simulink model "penddemo_disc"  (R2021a)
settings: Solver=ode8  StartTime=0  StopTime=inf  FixedStep=0.001  MaxStep=0.02  RelTol=1e-3  AbsTol=1e-6
undefined symbols (not defined in the file or in its folder): DiscIntNeverNeededParam
libraries: cstblocks x1
Description:
  | Inverted Pendulum with Animation
  | 
  | This example shows how to model an inverted pendulum.  The animation is created using MATLAB(R) Handle Graphics(R).  The animation block is a masked
  | S-function.  For more information, use the context menu to look under the Animation block's mask
  | and open the S-function for editing.
settings Model: ExtModeAutoUpdateStatusClock=off  Creator=The MathWorks, Inc.  LastModifiedBy=uidr9910
settings SolverCC: AutoScaleAbsTol=off  AlgebraicLoopSolver=TrustRegion
settings DataIOCC: ExternalInput=[]  InitialState=[]  SaveFormat=Array  SaveOutput=off  SaveTime=off
settings OptimizationCC: BlockReduction=off  BooleanDataType=off  ExpressionDepthLimit=2147483647  InitFltsAndDblsToZero=on  LifeSpan=inf
settings DebuggingCC: SaveWithParameterizedLinksMsg=none  UnderspecifiedInitializationDetection=Classic  MergeDetectMultiDrivingBlocksExec=none  SignalResolutionControl=TryResolveAllWithWarning  MultiTaskDSMMsg=warning  MultiTaskCondExecSysMsg=none  SigSpecEnsureSampleTimeMsg=none  FcnCallInpInsideContextMsg=warning  StateNameClashWarn=warning  SFUnexpectedBacktrackingDiag=warning  SFNoUnconditionalDefaultTransitionDiag=warning  SFExecutionAtInitializationDiag=none  SFMachineParentedDataDiag=warning  ArithmeticOperatorsInVariantConditions=warning
settings HardwareCC: ProdBitPerPointer=32  ProdBitPerSizeT=32  ProdBitPerPtrDiffT=32  ProdLargestAtomicFloat=None  ProdIntDivRoundTo=Undefined  ProdEndianess=Unspecified  ProdWordSize=32  ProdHWDeviceType=32-bit Generic  TargetUnknown=on
settings ModelReferenceCC: PropagateSignalLabelsOutOfModel=off
settings SFSimCC: SimUseLocalCustomCode=off  CustomCodeUndefinedFunction=UseInterfaceOnly
settings RTWCC: RTWUseLocalCustomCode=off
settings CodeAppCC: StateflowObjectComments=on
settings GRTTargetCC: TargetFcnLib=ansi_tfl_tmw.mat  TargetLangStandard=C89/C90 (ANSI)  CombineOutputUpdateFcns=off  GRTInterface=on
settings ConfigComp: CovMetricSettings=dw  CovSaveCumulativeToWorkspaceVar=on  CovSaveSingleToWorkspaceVar=on  CovExternalEMLEnable=off

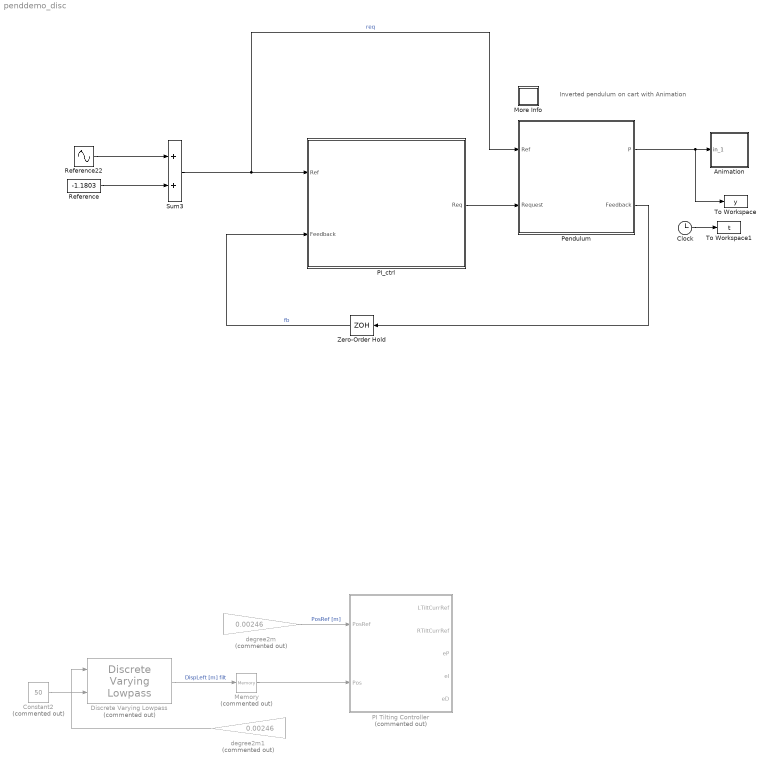
== system penddemo_disc ==
  note: Inverted pendulum on cart with Animation
  Animation : Subsystem  mask(Pendulum plot){RefBlock=Reference}
      mask prompts: RefBlock "DC reference signal block name:"
      mask help: Pendulum plot
      mask Help: Pendulum animation function using Handle graphics.
      mask Display: plot([-10 10],[0 0],[-2 -2 2 2],[0 1 1 0],[0 3],[1 5])
  Clock : Clock
  Constant2 : Constant  Commented=on  Value=50
  Discrete Varying Lowpass : cstblocks/Linear Parameter Varying/Discrete Varying Lowpass  Commented=on  N=1  w0=0.5  Ts=0.005
      settings: SourceProductBaseCode=CT
  Memory : Memory  Commented=on  InheritSampleTime=on
  More Info : Subsystem
      settings: OpenFcn=showExample('simulink_general/penddemoExample')
      mask Display: disp('?')
  PI Tilting Controller : MATLAB Function  Commented=on  TreatAsAtomicUnit=on  SystemSampleTime=5e-3
  PI_ctrl : Subsystem  mask{Kp=-10, Ki=0.05, Ts=0.005, Req_lim=15}
      mask prompts: Req_lim "Req_sat"
  Pendulum : Subsystem
  Reference : Constant  Value=-1.1803
  Reference22 : Sin  Amplitude=2  Frequency=0.5
  Sum3 : Sum  InputSameDT=on  SaturateOnIntegerOverflow=on  OutDataTypeStr=Inherit: Same as first input
  To Workspace : ToWorkspace  VariableName=y  SampleTime=0.1
  To Workspace1 : ToWorkspace  VariableName=t  SampleTime=0.1
  Zero-Order Hold : ZeroOrderHold  SampleTime=0.040
  degree2m : Gain  Commented=on  Gain=0.00246
  degree2m1 : Gain  Commented=on  Gain=0.00246
  wires:
  Pendulum/1(P) -> To Workspace/1, Animation/1(in_1)
  Clock/1 -> To Workspace1/1
  Reference/1 -> Sum3/2
  Reference22/1 -> Sum3/1
  degree2m/1 -> PI Tilting Controller/1(PosRef)  "PosRef [m]"
  Memory/1 -> PI Tilting Controller/2(Pos)
  Constant2/1 -> Discrete Varying Lowpass/2
  Discrete Varying Lowpass/1 -> Memory/1  "DispLeft [m] filt"
  degree2m1/1 -> Discrete Varying Lowpass/1
  Sum3/1 -> Pendulum/1(Ref), PI_ctrl/1(Ref)  "req"
  Pendulum/2(Feedback) -> Zero-Order Hold/1
  Zero-Order Hold/1 -> PI_ctrl/2(Feedback)  "fb"
  PI_ctrl/1(Req) -> Pendulum/2(Request)

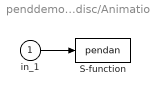
== system penddemo_disc/Animation ==
  in_1 : Inport
  S-function : S-Function  FunctionName=pendan  Parameters=RefBlock  SFunctionDeploymentMode=off  EnableBusSupport=off
      settings: DeleteFcn=pendan([],[],[],'DeleteBlock');
  wires:
  in_1/1 -> S-function/1

== system penddemo_disc/More Info ==

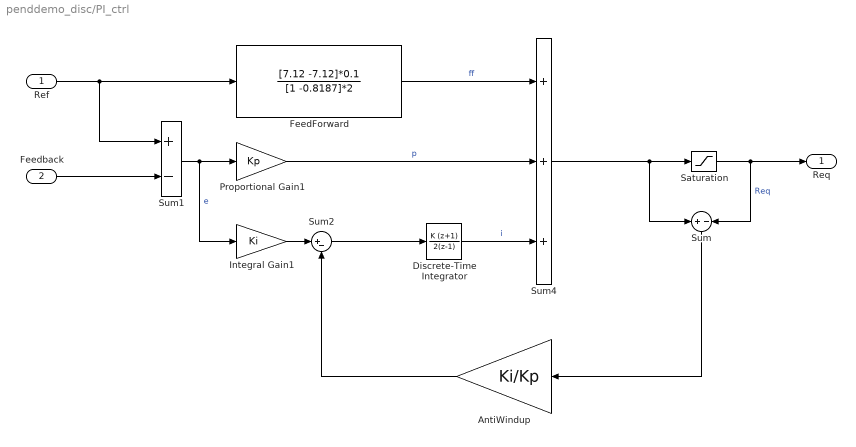
== system penddemo_disc/PI_ctrl ==
  Ref : Inport
  Feedback : Inport  Port=2
  AntiWindup : Gain  Gain=Ki/Kp  SaturateOnIntegerOverflow=on  OutDataTypeStr=Inherit: Same as input  ParamDataTypeStr=Inherit: Same as input
  Discrete-Time Integrator : DiscreteIntegrator  IntegratorMethod=Accumulation: Trapezoidal  gainval=Ts/5  SampleTime=-1  ICPrevOutput=DiscIntNeverNeededParam  ICPrevScaledInput=DiscIntNeverNeededParam
  FeedForward : DiscreteTransferFcn  Numerator=[7.12 -7.12]*0.1  Denominator=[1 -0.8187]*2  SampleTime=Ts
  Integral Gain1 : Gain  Gain=Ki  SaturateOnIntegerOverflow=on  OutDataTypeStr=Inherit: Same as input  ParamDataTypeStr=Inherit: Same as input
  Proportional Gain1 : Gain  Gain=Kp  SaturateOnIntegerOverflow=on  OutDataTypeStr=Inherit: Same as input  ParamDataTypeStr=Inherit: Same as input
  Saturation : Saturate  UpperLimit=Req_lim  LowerLimit=-Req_lim
  Sum : Sum  Inputs=+|-
  Sum1 : Sum  Inputs=+-  InputSameDT=on  SaturateOnIntegerOverflow=on  OutDataTypeStr=Inherit: Same as first input
  Sum2 : Sum  Inputs=|+-
  Sum4 : Sum  Inputs=+++  InputSameDT=on  SaturateOnIntegerOverflow=on  OutDataTypeStr=Inherit: Same as first input
  Req : Outport
  wires:
  Sum1/1 -> Integral Gain1/1, Proportional Gain1/1  "e"
  Saturation/1 -> Req/1, Sum/2  "Req"
  AntiWindup/1 -> Sum2/2
  Sum2/1 -> Discrete-Time Integrator/1
  Sum4/1 -> Sum/1, Saturation/1
  FeedForward/1 -> Sum4/1  "ff"
  Proportional Gain1/1 -> Sum4/2  "p"
  Integral Gain1/1 -> Sum2/1
  Sum/1 -> AntiWindup/1
  Discrete-Time Integrator/1 -> Sum4/3  "i"
  Feedback/1 -> Sum1/2
  Ref/1 -> Sum1/1, FeedForward/1

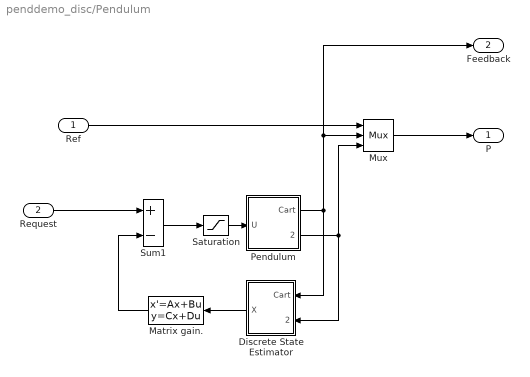
== system penddemo_disc/Pendulum ==
  Ref : Inport
  Request : Inport  Port=2
  Discrete State Estimator : Subsystem  mask(Pendulum Discrete state estimator){Ts=0.02}
      mask prompts: Ts "Sample time"
      mask help: Pendulum discrete state estimator
      mask Help: The states of the pendulum and cart system are the pendulum angle and angular velocity and cart position and velocity.  Since the sensors output the pendulum angle and cart position, this state estimator just does a one step difference calculation to get the velocities.
  Matrix gain. : StateSpace  A=[]  B=[]  C=[]  D=K  InitialCondition=0  mask(Matrix gain){K=[0 -18 -166.5 -15.2]*0.4}
      mask prompts: K "Gain matrix:"
      mask help: Matrix Gain:
      mask Help: Multiplies input vector by entered matrix to produce output vector.
      mask Display: disp('LQR')
  Mux : Mux  Inputs=3
  Pendulum : Subsystem  mask(Inverted pendulum on cart){Mcart=0.455/2, m=0.21*2, l=0.61/2, g=9.8}
      mask prompts: Mcart "Mass of cart (kg):"; m "Mass of pendulum (kg):"; l "Distance to pendulum center of mass(m):"; g "Acceleration of gravity (m/s^2):"
      mask help: Unmask and double-click to see dynamics
      mask Help: Nonlinear dynamics of inverted pendulum on cart.
  Saturation : Saturate  UpperLimit=10  LowerLimit=-10
  Sum1 : Sum  Inputs=+-  InputSameDT=on  SaturateOnIntegerOverflow=on  OutDataTypeStr=Inherit: Same as first input
  P : Outport
  Feedback : Outport  Port=2
  wires:
  Discrete State Estimator/1(X) -> Matrix gain./1
  Pendulum/2(Pendulum) -> Mux/3, Discrete State Estimator/2(Pendulum)
  Sum1/1 -> Saturation/1
  Ref/1 -> Mux/1
  Pendulum/1(Cart) -> Feedback/1, Mux/2, Discrete State Estimator/1(Cart)
  Saturation/1 -> Pendulum/1(U)
  Matrix gain./1 -> Sum1/2
  Request/1 -> Sum1/1
  Mux/1 -> P/1

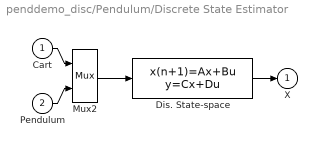
== system penddemo_disc/Pendulum/Discrete State Estimator ==
  Cart : Inport
  Pendulum : Inport  Port=2
  Dis. State-space : DiscreteStateSpace  A=zeros(2)  B=-eye(2)/Ts  C=[0 0; 1 0; 0 0; 0 1]  D=[1 0; 1/Ts 0; 0 1; 0 1/Ts]  SampleTime=Ts
  Mux2 : Mux  Inputs=2
  X : Outport  InitialOutput=0  VectorParamsAs1DForOutWhenUnconnected=off
  wires:
  Pendulum/1 -> Mux2/2
  Dis. State-space/1 -> X/1
  Cart/1 -> Mux2/1
  Mux2/1 -> Dis. State-space/1

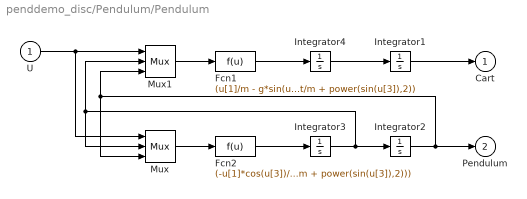
== system penddemo_disc/Pendulum/Pendulum ==
  U : Inport
  Fcn1 : Fcn  Expr=(u[1]/m - g*sin(u[3])*cos(u[3]) + l*power(u[2],2)*sin(u[3]))/(Mcart/m + power(sin(u[3]),2))
  Fcn2 : Fcn  Expr=(-u[1]*cos(u[3])/m + (Mcart+m)*g*sin(u[3])/m - l*power(u[2],2)*sin(u[3])*cos(u[3]))/(l*(Mcart/m + power(sin(u[3]),2)))
  Integrator{1..4} (4 alike) : Integrator
  Mux : Mux  Inputs=3
  Mux1 : Mux  Inputs=3
  Cart : Outport  InitialOutput=0  VectorParamsAs1DForOutWhenUnconnected=off
  Pendulum : Outport  Port=2  InitialOutput=0  VectorParamsAs1DForOutWhenUnconnected=off
  wires:
  Integrator1/1 -> Cart/1
  Fcn2/1 -> Integrator3/1
  Mux/1 -> Fcn2/1
  Mux1/1 -> Fcn1/1
  Fcn1/1 -> Integrator4/1
  Integrator4/1 -> Integrator1/1
  U/1 -> Mux1/1, Mux/1
  Integrator3/1 -> Integrator2/1, Mux1/2, Mux/2
  Integrator2/1 -> Pendulum/1, Mux1/3, Mux/3

== matlab function penddemo_disc/PI Tilting Controller ==
  data: PosRef input; LTiltCurrRef output; Pos input; RTiltCurrRef output; eP output; eI output; eD output
function [LTiltCurrRef, RTiltCurrRef,eP,eI,eD] = fcn(PosRef,Pos)
persistent uk1 ek1 ek2
if (isempty(uk1))
    uk1 = 0;
    ek1 = 0;
    ek2 = 0;
end

% +/- 0.076 m
pos_lim = 0.02;
imax = 10;

Kp =-9.4;
Ki = 0.01;
Kd = 0;

if (PosRef > pos_lim)
    PosRef = pos_lim;
end
if (PosRef <- pos_lim)
   PosRef = -pos_lim;
end

e = PosRef - Pos;


Du = Ki * e + Kp * (e - ek1) + Kd * (e - 2*ek1 + ek2);

eP = Kp*(e - ek1) ;
eI =  Ki*e ;
eD = Kd*(e - 2*ek1 + ek2);


u = uk1 + Du;

if (u >imax)
    u = imax;
end
if (u<-imax)
    u=-imax;
end

LTiltCurrRef =  u;
RTiltCurrRef =  -u;
uk1 = u;
ek1 = e;
ek2 = ek1;
